simulink model "BDamperOk"  (R2024b)
settings: Solver=FixedStepAuto  StartTime=0.0  StopTime=10.0  RelTol=1e-3  EnableMultiTasking=on
undefined symbols (not defined in the file): VDamperErrorHigh, VDamperErrorLow
libraries: simulink x8
settings Model: DataDictionary=Master_Dictionary.sldd  EnableAccessToBaseWorkspace=off  Creator=torni  LastModifiedBy=Will
settings OptimizationCC: DefaultParameterBehavior=Inlined  EnhancedBackFolding=on  PassReuseOutputArgsAs=Individual arguments  ZeroExternalMemoryAtStartup=off  ZeroInternalMemoryAtStartup=off  MaxStackSize=8192  OptimizeBlockOrder=speed  DifferentSizesBufferReuse=on  OptimizationCustomize=off  EfficientTunableParamExpr=on
settings DebuggingCC: ParameterTunabilityLossMsg=error
settings HardwareCC: ProdBitPerPointer=32  ProdBitPerSizeT=32  ProdBitPerPtrDiffT=32  ProdLargestAtomicInteger=Long  ProdLargestAtomicFloat=Double  ProdWordSize=32  ProdLongLongMode=on  ProdHWDeviceType=ARM Compatible->ARM Cortex-M
settings SFSimCC: MATLABDynamicMemAlloc=off
settings RTWCC: Description=Embedded Coder  SystemTargetFile=ert.tlc  HardwareBoard=STM32H7xx Based (Single-core)  TemplateMakefile=ert_default_tmf  Toolchain=GNU Tools for ARM Embedded Processors
settings CodeAppCC: ForceParamTrailComments=on  IgnoreCustomStorageClasses=off  OperatorAnnotations=on  SimulinkDataObjDesc=on  SFDataObjDesc=on  InsertBlockDesc=on
settings ERTTargetCC: TargetLangStandard=C99 (ISO)  CodeReplacementLibrary=ARM Cortex-M  ExtModeTransport=3  ExtModeStaticAlloc=on  ExtModeStaticAllocSize=2048  ExtModeMexFile=ext_xcp  ExtModeIntrfLevel=Level2 - Open

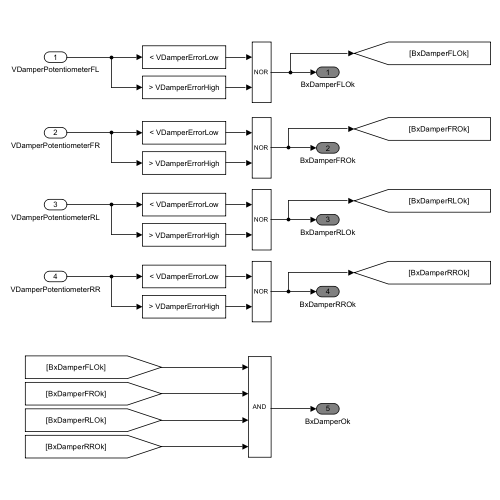
[thumbnail: Simulink's stored preview of the top-level diagram]
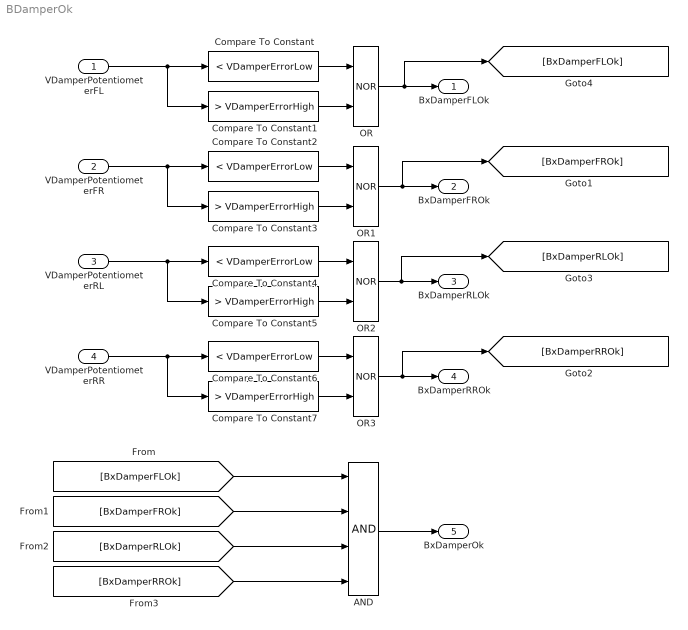
== system BDamperOk ==
  VDamperPotentiometerFL : Inport  OutDataTypeStr=double
  "VDamperPotentiometerFR " : Inport  Port=2  OutDataTypeStr=double
  VDamperPotentiometerRL : Inport  Port=3  OutDataTypeStr=double
  VDamperPotentiometerRR : Inport  Port=4  OutDataTypeStr=double
  AND : Logic  Inputs=4  AllPortsSameDT=off  OutDataTypeStr=boolean
  Compare To Constant{,2,4,6} (4 alike) : simulink/Logic and Bit Operations/Compare To Constant  relop=<  const=VDamperErrorLow  OutDataTypeStr=boolean
  Compare To Constant{1,3,5,7} (4 alike) : simulink/Logic and Bit Operations/Compare To Constant  relop=>  const=VDamperErrorHigh  OutDataTypeStr=boolean
  OR{,1..3} (4 alike) : Logic  Operator=NOR  AllPortsSameDT=off  OutDataTypeStr=boolean
  BxDamperFLOk : Outport  OutDataTypeStr=boolean  VectorParamsAs1DForOutWhenUnconnected=off
  BxDamperFROk : Outport  Port=2  OutDataTypeStr=boolean  VectorParamsAs1DForOutWhenUnconnected=off
  BxDamperRLOk : Outport  Port=3  OutDataTypeStr=boolean  VectorParamsAs1DForOutWhenUnconnected=off
  BxDamperRROk : Outport  Port=4  OutDataTypeStr=boolean  VectorParamsAs1DForOutWhenUnconnected=off
  BxDamperOk : Outport  Port=5  OutDataTypeStr=boolean  VectorParamsAs1DForOutWhenUnconnected=off
  wires:
  Compare To Constant1/1 -> OR/2
  Compare To Constant/1 -> OR/1
  OR3/1 -> [BxDamperRROk], BxDamperRROk/1
  VDamperPotentiometerFL/1 -> Compare To Constant1/1, Compare To Constant/1
  OR/1 -> [BxDamperFLOk], BxDamperFLOk/1
  OR1/1 -> [BxDamperFROk], BxDamperFROk/1
  "VDamperPotentiometerFR "/1 -> Compare To Constant2/1, Compare To Constant3/1
  Compare To Constant2/1 -> OR1/1
  Compare To Constant3/1 -> OR1/2
  Compare To Constant5/1 -> OR2/2
  Compare To Constant4/1 -> OR2/1
  VDamperPotentiometerRL/1 -> Compare To Constant5/1, Compare To Constant4/1
  OR2/1 -> [BxDamperRLOk], BxDamperRLOk/1
  VDamperPotentiometerRR/1 -> Compare To Constant6/1, Compare To Constant7/1
  Compare To Constant6/1 -> OR3/1
  Compare To Constant7/1 -> OR3/2
  [BxDamperRROk] -> AND/4
  [BxDamperRLOk] -> AND/3
  [BxDamperFROk] -> AND/2
  [BxDamperFLOk] -> AND/1
  AND/1 -> BxDamperOk/1
